simulink model "BBW_ABS_2023HT65255"  (R2023a)
settings: Solver=VariableStepAuto  StartTime=0.0  StopTime=25  RelTol=1e-3
values from neighbouring files (symbols this model uses):
  g = 9.81    [BBW_ABS_Script_2023HT65255.m]
  I = 4    [BBW_ABS_Script_2023HT65255.m]
  m = 75    [BBW_ABS_Script_2023HT65255.m]
  R = 1.25    [BBW_ABS_Script_2023HT65255.m]
undefined symbols (not defined in the file or in its folder): DiscIntNeverNeededParam
settings Model: Creator=sidhe  LastModifiedBy=sidhe
settings OptimizationCC: DefaultParameterBehavior=Inlined  UseDivisionForNetSlopeComputation=on  GainParamInheritBuiltInType=on  UseFloatMulNetSlope=on  InlineInvariantSignals=on  PassReuseOutputArgsAs=Individual arguments  ZeroExternalMemoryAtStartup=off  ZeroInternalMemoryAtStartup=off  NoFixptDivByZeroProtection=on  EfficientFloat2IntCast=on  LifeSpan=1  OptimizeBlockOrder=speed  DifferentSizesBufferReuse=on  EfficientTunableParamExpr=on
settings DebuggingCC: MultiTaskDSMMsg=warning  ParameterDowncastMsg=warning  ParameterOverflowMsg=warning  ParameterTunabilityLossMsg=error  UniqueDataStoreMsg=warning
settings HardwareCC: ProdBitPerPointer=32  ProdBitPerSizeT=32  ProdBitPerPtrDiffT=32  ProdWordSize=32  ProdLongLongMode=on  ProdHWDeviceType=Intel->x86-32 (Windows32)
settings SFSimCC: MATLABDynamicMemAlloc=off
settings RTWCC: Description=Embedded Coder  SystemTargetFile=ert.tlc  TemplateMakefile=ert_default_tmf
settings CodeAppCC: ForceParamTrailComments=on  IgnoreCustomStorageClasses=off  OperatorAnnotations=on  SimulinkDataObjDesc=on  SFDataObjDesc=on  CustomSymbolStrGlobalVar=rt$N$M  CustomSymbolStrType=$N$M  CustomSymbolStrFcn=$N$M$F  CustomSymbolStrMacro=$N$M  InsertBlockDesc=on
settings ERTTargetCC: TargetLangStandard=C99 (ISO)  GenerateSampleERTMain=on  IncludeMdlTerminateFcn=off  CombineSignalStateStructs=on  SuppressErrorStatus=on  SupportAbsoluteTime=off  SupportNonFinite=off  SupportComplex=off  InlinedParameterPlacement=NonHierarchical  ERTCustomFileTemplate=example_file_process.tlc  ERTFilePackagingFormat=CompactWithDataFile

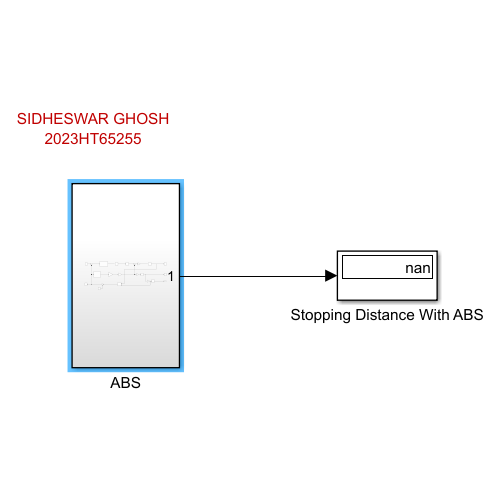
[thumbnail: Simulink's stored preview of the top-level diagram]
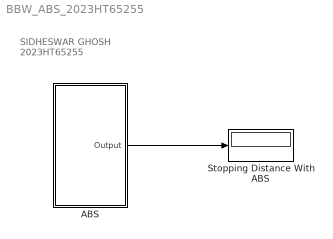
== system BBW_ABS_2023HT65255 ==
  note: SIDHESWAR GHOSH
      | 2023HT65255
  ABS : Subsystem
  Stopping Distance With ABS : Display
  wires:
  ABS/1(Output) -> Stopping Distance With ABS/1

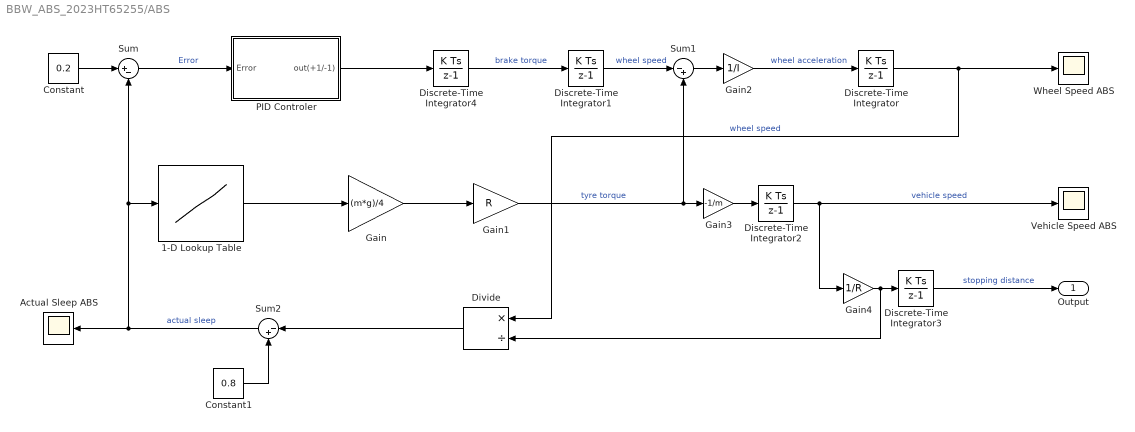
== system BBW_ABS_2023HT65255/ABS ==
  1-D Lookup Table : Lookup_n-D  NumberOfTableDimensions=1  BreakpointsForDimension1=|  Table=|  InternalRulePriority=Speed  RndMeth=Simplest
      BreakpointsForDimension1=|
      | [0
      | 0.05
      | 0.1
      | 0.15
      | 0.2
      | 0.25
      | 0.35
      | 0.4
      | 0.45
      | 0.5
      | 0.55
      | 0.6
      | 0.65
      | 0.7
      | 0.75
      | 0.8
      | 0.85
      | 0.9
      | 0.95
      | 1
      | ]
      Table=|
      | tanh([0
      | 0.4
      | 0.8
      | 0.97
      | 1
      | 0.98
      | 0.96
      | 0.94
      | 0.92
      | 0.9
      | 0.855
      | 0.83
      | 0.81
      | 0.79
      | 0.77
      | 0.75
      | 0.73
      | 0.72
      | 0.71
      | 0.7
      | ])
  Actual Sleep ABS : Scope
  Constant : Constant  Value=0.2  SampleTime=-1
  Constant1 : Constant  Value=0.8  SampleTime=-1
  Discrete-Time Integrator{,1..4} (5 alike) : DiscreteIntegrator  SampleTime=0.001  ICPrevOutput=DiscIntNeverNeededParam  ICPrevScaledInput=DiscIntNeverNeededParam
  Divide : Product  Inputs=*/
  Gain : Gain  Gain=(m*g)/4
  Gain1 : Gain  Gain=R
  Gain2 : Gain  Gain=1/I
  Gain3 : Gain  Gain=-1/m
  Gain4 : Gain  Gain=1/R
  PID Controler : Subsystem
  Sum : Sum  Inputs=|+-
  Sum1 : Sum  Inputs=|-+
  Sum2 : Sum  Inputs=|-+
  Vehicle Speed ABS : Scope
  Wheel Speed ABS : Scope
  Output : Outport
  wires:
  Gain4/1 -> Discrete-Time Integrator3/1, Divide/2
  Gain1/1 -> Gain3/1, Sum1/2  "tyre torque"
  PID Controler/1(out(+1/-1)) -> Discrete-Time Integrator4/1
  Divide/1 -> Sum2/1
  Sum/1 -> PID Controler/1(Error)  "Error"
  Constant/1 -> Sum/1
  1-D Lookup Table/1 -> Gain/1
  Discrete-Time Integrator2/1 -> Gain4/1, Vehicle Speed ABS/1  "vehicle speed"
  Discrete-Time Integrator4/1 -> Discrete-Time Integrator1/1  "brake torque"
  Gain2/1 -> Discrete-Time Integrator/1  "wheel acceleration"
  Sum2/1 -> Actual Sleep ABS/1, 1-D Lookup Table/1, Sum/2  "actual sleep"
  Gain/1 -> Gain1/1
  Discrete-Time Integrator3/1 -> Output/1  "stopping distance"
  Gain3/1 -> Discrete-Time Integrator2/1
  Discrete-Time Integrator/1 -> Divide/1, Wheel Speed ABS/1  "wheel speed"
  Constant1/1 -> Sum2/2
  Sum1/1 -> Gain2/1
  Discrete-Time Integrator1/1 -> Sum1/1  "wheel speed"

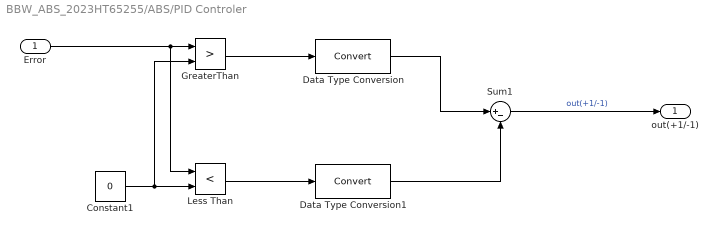
== system BBW_ABS_2023HT65255/ABS/PID Controler ==
  Error : Inport
  Constant1 : Constant  Value=0  SampleTime=-1
  Data Type Conversion : DataTypeConversion  SaturateOnIntegerOverflow=off  RndMeth=Floor
  Data Type Conversion1 : DataTypeConversion  SaturateOnIntegerOverflow=off  RndMeth=Floor
  GreaterThan : RelationalOperator  Operator=>  OutDataTypeStr=boolean  RndMeth=Simplest  InputSameDT=off
  Less Than : RelationalOperator  Operator=<  OutDataTypeStr=boolean  RndMeth=Simplest  InputSameDT=off
  Sum1 : Sum  Inputs=|+-
  out(+1/-1) : Outport
  wires:
  Error/1 -> Less Than/1, GreaterThan/1
  Sum1/1 -> out(+1/-1)/1  "out(+1/-1)"
  Data Type Conversion1/1 -> Sum1/2
  Less Than/1 -> Data Type Conversion1/1
  Constant1/1 -> GreaterThan/2, Less Than/2
  GreaterThan/1 -> Data Type Conversion/1
  Data Type Conversion/1 -> Sum1/1
